simulink model "kbk3PEMANASSOLDER2"  (R2014a)
settings: Solver=ode3  StartTime=0.0  StopTime=200  RelTol=1e-3
libraries: arduino_io_lib x4
settings Model: Creator=Gadis  LastModifiedBy=Gadis

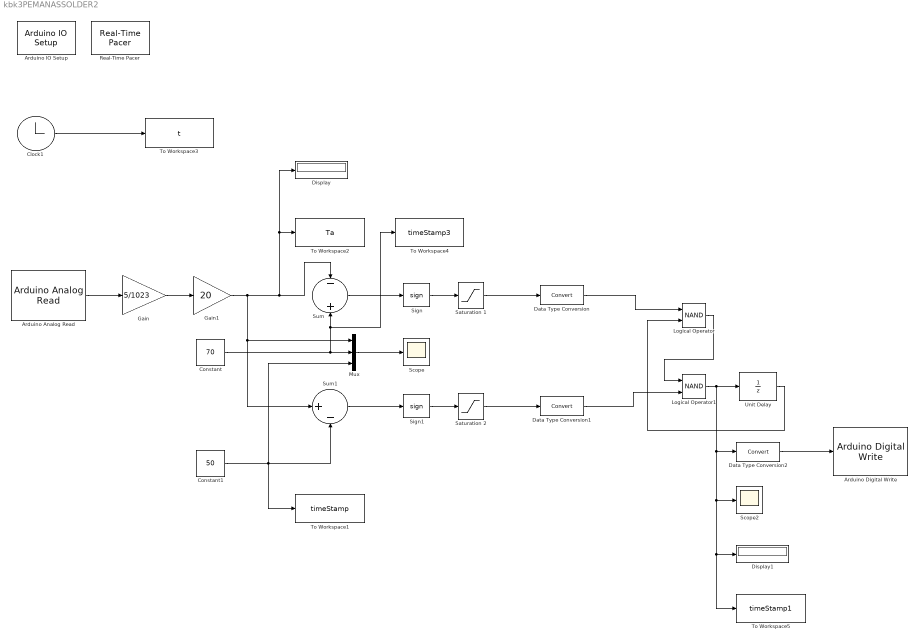
== system kbk3PEMANASSOLDER2 ==
  Arduino Analog Read : arduino_io_lib/Arduino Analog Read  arduinoVar=Temporary arduino variable: Arduino1  arduinoPin=0  T=0.2
  Arduino Digital Write : arduino_io_lib/Arduino Digital Write  arduinoVar=Temporary arduino variable: Arduino1  arduinoPin=3  T=0.2
  Arduino IO Setup : arduino_io_lib/Arduino IO Setup  Priority=3  arduinoVar=Temporary arduino variable: Arduino1  workspaceVarName=a  comPort=COM21
  Clock1 : Clock
  Constant : Constant  Value=70
  Constant1 : Constant  Value=50
  Data Type Conversion : DataTypeConversion
  Data Type Conversion1 : DataTypeConversion
  Data Type Conversion2 : DataTypeConversion
  Display : Display
  Display1 : Display
  Gain : Gain  Gain=5/1023
  Gain1 : Gain  Gain=20
  Logical Operator : Logic  Operator=NAND  IconShape=distinctive  AllPortsSameDT=off  OutDataTypeStr=boolean
  Logical Operator1 : Logic  Operator=NAND  IconShape=distinctive  AllPortsSameDT=off  OutDataTypeStr=boolean
  Mux : Mux  Inputs=3
  Real-Time Pacer : arduino_io_lib/Real-Time Pacer  simTimePerRealTime=1
  Saturation 1 : Saturate  UpperLimit=1  LowerLimit=0
  Saturation 2 : Saturate  UpperLimit=1  LowerLimit=0
  Scope : Scope
      settings: YMin=47  YMax=70
  Scope2 : Scope
      settings: YMin=1  YMax=1  SaveName=ScopeData2
  Sign : Signum
  Sign1 : Signum
  Sum : Sum  Inputs=-+
  Sum1 : Sum  Inputs=|+-
  To Workspace1 : ToWorkspace  VariableName=timeStamp  SampleTime=-1
  To Workspace2 : ToWorkspace  VariableName=Ta  SaveFormat=Timeseries  SampleTime=-1
  To Workspace3 : ToWorkspace  VariableName=t  SampleTime=-1
  To Workspace4 : ToWorkspace  VariableName=timeStamp3  SampleTime=-1
  To Workspace5 : ToWorkspace  VariableName=timeStamp1  SampleTime=-1
  Unit Delay : UnitDelay  SampleTime=-1
  wires:
  Arduino Analog Read/1 -> Gain/1
  Gain/1 -> Gain1/1
  Sign/1 -> Saturation 1/1
  Sum/1 -> Sign/1
  Clock1/1 -> To Workspace3/1
  Saturation 1/1 -> Data Type Conversion/1
  Sign1/1 -> Saturation 2/1
  Sum1/1 -> Sign1/1
  Saturation 2/1 -> Data Type Conversion1/1
  Constant1/1 -> Mux/3, To Workspace1/1, Sum1/2
  Gain1/1 -> Mux/1, Sum1/1, Sum/1, Display/1, To Workspace2/1
  Constant/1 -> To Workspace4/1, Sum/2, Mux/2
  Mux/1 -> Scope/1
  Data Type Conversion/1 -> Logical Operator/1
  Data Type Conversion1/1 -> Logical Operator1/2
  Logical Operator/1 -> Logical Operator1/1
  Logical Operator1/1 -> To Workspace5/1, Display1/1, Scope2/1, Data Type Conversion2/1, Unit Delay/1
  Data Type Conversion2/1 -> Arduino Digital Write/1
  Unit Delay/1 -> Logical Operator/2
